simulink model "test_kalman_scaling"  (R2024a)
settings: Solver=FixedStepAuto  StartTime=0.0  StopTime=4e-4  FixedStep=8e-9  RelTol=1e-3
values from neighbouring files (symbols this model uses):
  A1 = [0,                  1,  0, 0,   0, 0 ... (first row only)    [three_axis_plant_ver_0_init.m]
  A2 = [0,                  1,  0, 0,   0, 0 ... (first row only)    [three_axis_plant_ver_0_init.m]
  B1 = [0; p.C_f/p.m; 0; p.C_f_xz/p.m; 0; p.C_f_xy/p.m;]    [three_axis_plant_ver_0_init.m]
  C1 = [p.C_el_x,  0,         p.C_el_xz,    0, p.C_el_xy, 0;       0,         p.C_el_x,          0,    0,         0, 0;       p.C_el_zx,        0,   p.C_el_z,    0,    p.C_el_zy, 0]    [three_axis_plant_ver_0_init.m]
  eff_fun = @(V) cos(eff_w.*V.^2)./(eff_m*V.^4 + eff_n) + eff_p    [three_axis_plant_ver_0_init.m]
  G1 = [0 0 0; 1/p.m 0 0; 0 0 0; 0 1/p.m 0; 0 0 0; 0 0 1/p.m]    [three_axis_plant_ver_0_init.m]
  t_off = 2*T_max +(t_on + 100*(2*pi/abs(p.Omega_ip)))    [three_axis_plant_ver_0_init.m]
  t_on = 0*2*T_max*0.01    [three_axis_plant_ver_0_init.m]
undefined symbols (not defined in the file or in its folder): clqr, k, lqg, p, xc7z020clg400
libraries: hdlSSR x61, hdlBasic x40, simulink x10, vmcUtilities x1
(part 1 of 2)
settings Model: Creator=berndorfer
settings DebuggingCC: UnconnectedInputMsg=warning  UnconnectedOutputMsg=warning  UnconnectedLineMsg=warning
settings ModelReferenceCC: EnableRefExpFcnMdlSchedulingChecks=on
settings RTWCC: GPUComputeCapability=3.5  DLArmComputeVersion=19.05

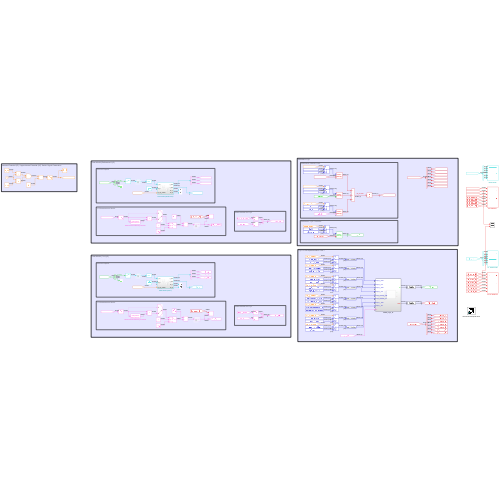
[thumbnail: Simulink's stored preview of the top-level diagram]
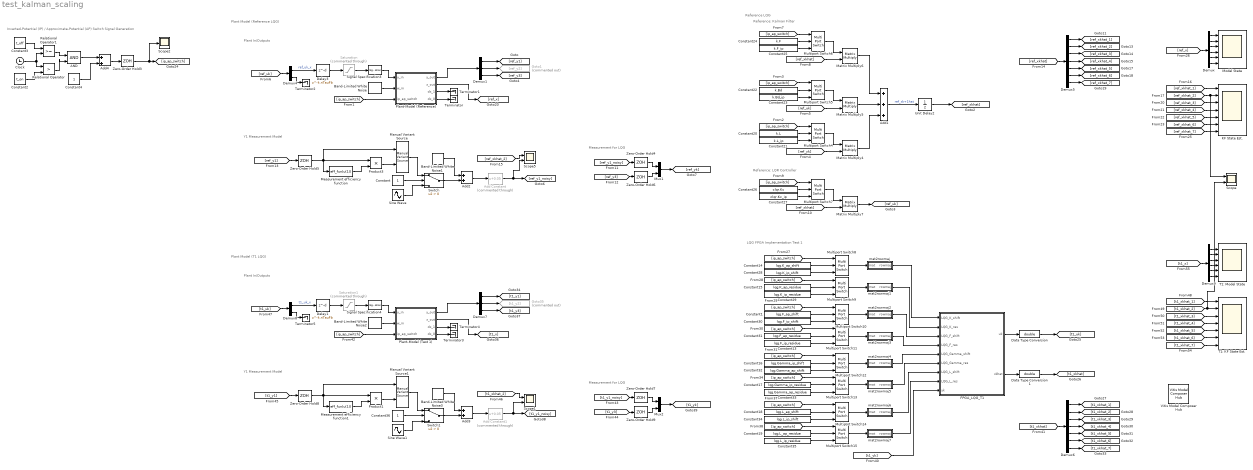
== system test_kalman_scaling ==
  note: LQG FPGA Implementation Test 1
  note: Plant In/Outputs
  note: Y1 Measurement Model
  note: Measurement for LQG
  note: Reference: LQR Controller
  note: Reference: Kalman Filter
  note: Reference LQG
  note: Plant Model (Reference LQG)
  note: Inverted-Potential (IP) / Approximate-Potential (AP) Switch Signal Generation
  note: Y1 Measurement Model
  note: Plant Model (T1 LQG)
  note: Plant In/Outputs
  note: Measurement for LQG
  AND : Logic  IconShape=distinctive  AllPortsSameDT=off  OutDataTypeStr=boolean
  Add Constant : Bias  Commented=through  Bias=0.05  SaturateOnIntegerOverflow=off
  Add Constant1 : Bias  Commented=through  Bias=0.05  SaturateOnIntegerOverflow=off
  Add1 : Sum  Inputs=+++
  Add2 : Sum
  Add3 : Sum
  Add4 : Sum
  Band-Limited White Noise : simulink/Sources/Band-Limited White Noise  Cov=P_W  Ts=p.Ts  seed=[23341; 896784; 46532]
  Band-Limited White Noise1 : simulink/Sources/Band-Limited White Noise  Cov=P_V  Ts=1/k.f_samp  seed=[73341]
  Band-Limited White Noise2 : simulink/Sources/Band-Limited White Noise  Cov=P_W  Ts=p.Ts  seed=[23341; 896784; 46532]
  Band-Limited White Noise3 : simulink/Sources/Band-Limited White Noise  Cov=P_V  Ts=1/k.f_samp  seed=[73341]
  Clock : Clock
  Constant : Constant
  Constant1 : Constant  Value=lqg.F_ap_shift  SampleTime=p.Ts
  Constant13 : Constant  Value=lqg.F_ip_residue  SampleTime=p.Ts
  Constant14 : Constant  Value=lqg.K_ap_shift  SampleTime=p.Ts
  Constant15 : Constant  Value=lqg.K_ap_residue  VectorParams1D=off  SampleTime=p.Ts
  Constant16 : Constant  Value=lqg.Gamma_ip_shift  SampleTime=p.Ts
  Constant17 : Constant  Value=lqg.Gamma_ip_residue  SampleTime=p.Ts
  Constant18 : Constant  Value=lqg.L_ap_shift  SampleTime=p.Ts
  Constant19 : Constant  Value=lqg.L_ap_residue  SampleTime=p.Ts
  Constant2 : Constant  Value=t_on
  Constant20 : Constant  Value=k.L  SampleTime=k.Ts
  Constant21 : Constant  Value=k.L_ip  SampleTime=k.Ts
  Constant22 : Constant  Value=k.Bd  SampleTime=k.Ts
  Constant23 : Constant  Value=k.Bd_ip  SampleTime=k.Ts
  Constant24 : Constant  Value=k.F  SampleTime=k.Ts
  Constant25 : Constant  Value=k.F_ip  SampleTime=k.Ts
  Constant26 : Constant  Value=clqr.Kc  SampleTime=k.Ts
  Constant27 : Constant  Value=clqr.Kc_ip  SampleTime=k.Ts
  Constant28 : Constant  Value=lqg.K_ip_shift  SampleTime=p.Ts
  Constant29 : Constant  Value=lqg.K_ip_residue  VectorParams1D=off  SampleTime=p.Ts
  Constant3 : Constant  Value=t_off
  Constant30 : Constant  Value=lqg.F_ip_shift  SampleTime=p.Ts
  Constant31 : Constant  Value=lqg.F_ap_residue  SampleTime=p.Ts
  Constant32 : Constant  Value=lqg.Gamma_ap_shift  SampleTime=p.Ts
  Constant33 : Constant  Value=lqg.Gamma_ap_residue  SampleTime=p.Ts
  Constant34 : Constant  Value=lqg.L_ip_shift  SampleTime=p.Ts
  Constant35 : Constant  Value=lqg.L_ip_residue  SampleTime=p.Ts
  Constant36 : Constant
  Constant4 : Constant
  Data Type Conversion : DataTypeConversion  OutDataTypeStr=double  SaturateOnIntegerOverflow=off  RndMeth=Floor
  Data Type Conversion1 : DataTypeConversion  OutDataTypeStr=double  SaturateOnIntegerOverflow=off  RndMeth=Floor
  Delay1 : Delay  DelayLength=k.nTauFb  SampleTime=k.Ts
  Delay3 : Delay  DelayLength=k.nTauFb  SampleTime=k.Ts
  Demux : Demux  Outputs=6
  Demux1 : Demux  Outputs=3
  Demux4 : Demux  Outputs=2
  Demux5 : Demux  Outputs=7
  Demux6 : Demux  Outputs=7
  Demux7 : Demux  Outputs=3
  Demux8 : Demux  Outputs=2
  Demux9 : Demux  Outputs=6
  FPGA_LQG_T1 : Subsystem
  Goto1 : Goto  Commented=on  GotoTag=ref_y2
  Goto35 : Goto  Commented=on  GotoTag=t1_y2
  KF State Est. : Scope  NumInputPorts=7
  Manual Variant Source : simulink/Signal Routing/Manual Variant Source  NumChoices=2  LabelModeActiveChoice=V_2
  Manual Variant Source1 : simulink/Signal Routing/Manual Variant Source  NumChoices=2  LabelModeActiveChoice=V_2
  Matrix Multiply{4..7} (4 alike) : Product  Multiplication=Matrix(*)
  Measurement efficiency function : MATLABFcn  MATLABFcn=eff_fun(u(1))
  Measurement efficiency function1 : MATLABFcn  MATLABFcn=eff_fun(u(1))
  Model State : Scope  NumInputPorts=6
  Multiport Switch{4..15} (12 alike) : MultiPortSwitch  Inputs=2  DiagnosticForDefault=Warning  SaturateOnIntegerOverflow=off  InputSameDT=off
  Mux1 : Mux  Inputs=2
  Mux2 : Mux  Inputs=2
  Plant-Model (Reference) : Subsystem
  Plant-Model (Test 1) : Subsystem
  Product1 : Product
  Product3 : Product
  Relational Operator : RelationalOperator  Operator=>  OutDataTypeStr=boolean  RndMeth=Simplest  InputSameDT=off
  Relational Operator1 : RelationalOperator  OutDataTypeStr=boolean  RndMeth=Simplest  InputSameDT=off
  Saturation : Saturate  Commented=through  UpperLimit=5  LowerLimit=-5
  Saturation1 : Saturate  Commented=through  UpperLimit=5  LowerLimit=-5
  Scope : Scope  NumInputPorts=2
  Scope1 : Scope  NumInputPorts=2
  Scope2 : Scope
  Scope5 : Scope  NumInputPorts=2
  Signal Specification3 : SignalSpecification  Dimensions=1
  Signal Specification4 : SignalSpecification  Dimensions=1
  Sine Wave : Sin  Amplitude=0.2  Frequency=2*pi*160e3  SampleTime=0
  Sine Wave1 : Sin  Amplitude=0.2  Frequency=2*pi*160e3  SampleTime=0
  Switch : Switch  Criteria=u2 > Threshold  SaturateOnIntegerOverflow=off  InputSameDT=off
  Switch1 : Switch  Criteria=u2 > Threshold  SaturateOnIntegerOverflow=off  InputSameDT=off
  T1: KF State Est. : Scope  NumInputPorts=7
  T1: Model State : Scope  NumInputPorts=6
  Terminator{,1..5} (6 alike) : Terminator
  Unit Delay2 : UnitDelay  InitialCondition=zeros(k.n_x,1)  SampleTime=k.Ts  HasFrameUpgradeWarning=on
  Vitis Model Composer Hub : vmcUtilities/Vitis Model Composer Hub  Tag=genX  CodeGeneration=off  SubsystemName=FPGA_LQG_T1  CompilationType=HDLCompilation  SubsystemType=HDLNode  ExportTypeV2=IP Catalog  StartColumn=1  NumberOfColumns=1  TargetDirectory=./netlist_lqg_t1  exportDesign=on  analyzeDesign=off  validateDesignOnHw=off  ExportType=AI Engines  IpVendor=xilinx.com  IpLibrary=hls  IpVersion=1.0  IpHWLanguage=Verilog  AieCompilerOptions={}  AieSimulatorOptions={}  CreateTestbench=off  TestbenchStackSize=10  RunRtlSim=off  RunCSim=off  RunAieSim=off  AieSimTimeout=50000  RunAieSimProfiling=off  LaunchVitisAnalyzer=off  PlotOutput=off  RunX86Sim=off  X86SimTimeout=10  GenHwImage=off  GenLibadfXo=on  GenHwValidationCode=off  PlatformType=Not Specified  HwSystemType=Baremetal  HwValidationTarget=hw  ProjDevice=xc7z020clg400-2  ProjDevicePart=xc7z020clg400-2  AIEType=None  SamplePeriod=-1  ClockFrequency=200  DataPathParallelism=1  xilinxfamily=zynq  part=xc7z020  speed=-2  package=clg400  directory=./code/ip/FPGA_LQG_T1/src  testbench=off  incr_netlist=off  synthesis_tool=Vivado  clock_wrapper=Clock Enables  dbl_ovrd=According to Block Masks  dcm_input_clock_period=10  sysclk_period=64  simulink_period=64e-9  eval_field=0  IPInfoJsonString="{\"DUTSubsystemName\":\"FPGA_LQG_T1\",\"HDLSubsystem\":{\"SubsystemName\":\"FPGA_LQG_T1\",\"IPName\":\"FPGA_LQG_Scaling_Test\",\"IPLibrary\":\"VMC\",\"IPVendor\":\"ACIN\",\"IPVersion\":\"1.0\",\"TargetDirectory\":\"./netlist_lqg_t1\",\"SubsystemDir\":\"./netlist_lqg_t1/ip/FPGA_LQG_T1\",\"FreqHz\":\"15625000\"},\"SubsystemTag\":\"HDLNode\"}"  LogFileName=/home/user/host_home/work/acin/projects/universal_lqg/lqg-fp7-firmware/matlab/netlist_lqg_t1/model_composer.log  NThreads=4  IPConfigFile=/tmp/vmctmp-user/13/ipconfig.json
  Zero-Order Hold3 : ZeroOrderHold  SampleTime=p.Ts
  Zero-Order Hold{4,6..7,9} (4 alike) : ZeroOrderHold  SampleTime=1/k.f_samp
  Zero-Order Hold5 : ZeroOrderHold  SampleTime=p.Ts
  Zero-Order Hold8 : ZeroOrderHold  SampleTime=p.Ts
  mat2rowmaj : Subsystem
  mat2rowmaj1 : Subsystem
  mat2rowmaj2 : Subsystem
  mat2rowmaj3 : Subsystem
  mat2rowmaj4 : Subsystem
  mat2rowmaj5 : Subsystem
  mat2rowmaj6 : Subsystem
  mat2rowmaj7 : Subsystem
  wires:
  Band-Limited White Noise/1 -> Plant-Model (Reference)/2(w_in)
  [ip_ap_switch] -> Plant-Model (Reference)/3(ip_ap_switch)
  AND/1 -> Add4/1
  Constant2/1 -> Relational Operator/2
  Clock/1 -> Relational Operator/1, Relational Operator1/2
  Relational Operator1/1 -> AND/1
  Add4/1 -> Zero-Order Hold3/1
  Relational Operator/1 -> AND/2
  Constant3/1 -> Relational Operator1/1
  Constant4/1 -> Add4/2
  Plant-Model (Reference)/1(y_out) -> Demux1/1
  Demux1/3 -> [ref_y3]
  Demux1/1 -> [ref_y1]
  Plant-Model (Reference)/2(x_out) -> [ref_x]
  Measurement efficiency function/1 -> Product3/2
  Sine Wave/1 -> Switch/3
  Switch/1 -> Add2/2
  Product3/1 -> Manual Variant Source/2
  Add2/1 -> Add Constant/1
  Constant/1 -> Switch/2
  Band-Limited White Noise1/1 -> Add2/1
  Add Constant/1 -> Scope5/2, [ref_y1_noisy]
  Zero-Order Hold5/1 -> Measurement efficiency function/1, Manual Variant Source/1, Product3/1
  [ref_y1] -> Zero-Order Hold5/1
  Signal Specification3/1 -> Plant-Model (Reference)/1(u_in)
  Saturation/1 -> Signal Specification3/1
  Delay3/1 -> Saturation/1
  Demux4/1 -> Delay3/1  "ref_uk_x"
  Demux1/2 -> Goto1/1
  Zero-Order Hold3/1 -> Scope2/1, [ip_ap_switch]
  Plant-Model (Reference)/4(dx_0) -> Terminator/1
  Plant-Model (Reference)/3(dx_1) -> Terminator1/1
  Constant20/1 -> Multiport Switch4/2
  [ip_ap_switch] -> Multiport Switch4/1
  Constant21/1 -> Multiport Switch4/3
  [ip_ap_switch] -> Multiport Switch5/1
  Constant22/1 -> Multiport Switch5/2
  Constant23/1 -> Multiport Switch5/3
  Multiport Switch4/1 -> Matrix Multiply4/1
  [ref_yk] -> Matrix Multiply4/2
  Multiport Switch5/1 -> Matrix Multiply5/1
  [ref_uk] -> Matrix Multiply5/2
  Constant24/1 -> Multiport Switch6/2
  Constant25/1 -> Multiport Switch6/3
  Multiport Switch6/1 -> Matrix Multiply6/1
  [ip_ap_switch] -> Multiport Switch6/1
  [ref_xkhat] -> Matrix Multiply6/2
  Matrix Multiply5/1 -> Add1/2
  Matrix Multiply6/1 -> Add1/1
  Matrix Multiply4/1 -> Add1/3
  Add1/1 -> Unit Delay2/1  "ref_xk+1hat"
  Unit Delay2/1 -> [ref_xkhat]
  Demux4/2 -> Terminator2/1
  [ref_uk] -> Demux4/1
  Constant26/1 -> Multiport Switch7/2
  Constant27/1 -> Multiport Switch7/3
  [ip_ap_switch] -> Multiport Switch7/1
  Multiport Switch7/1 -> Matrix Multiply7/1
  [ref_xkhat] -> Matrix Multiply7/2
  Matrix Multiply7/1 -> [ref_uk]
  [ref_y1_noisy] -> Zero-Order Hold4/1
  [ref_y3] -> Zero-Order Hold6/1
  Zero-Order Hold4/1 -> Mux1/1
  Zero-Order Hold6/1 -> Mux1/2
  Mux1/1 -> [ref_yk]
  Manual Variant Source/1 -> Switch/1
  [ref_xkhat] -> Demux5/1
  Demux5/1 -> [ref_xkhat_1]
  Demux5/2 -> [ref_xkhat_2]
  Demux5/3 -> [ref_xkhat_3]
  Demux5/4 -> [ref_xkhat_4]
  Demux5/5 -> [ref_xkhat_5]
  Demux5/6 -> [ref_xkhat_6]
  Demux5/7 -> [ref_xkhat_7]
  [ref_xkhat_2] -> Scope5/1
  [ref_xkhat_1] -> KF State Est./1
  [ref_xkhat_2] -> Scope/1, KF State Est./2
  [ref_xkhat_3] -> KF State Est./3
  [ref_xkhat_4] -> KF State Est./4
  [ref_xkhat_5] -> KF State Est./5
  [ref_xkhat_6] -> KF State Est./6
  [ref_xkhat_7] -> KF State Est./7
  Demux/5 -> Model State/5
  Demux/4 -> Model State/4
  Demux/1 -> Model State/1
  Demux/3 -> Model State/3
  Demux/2 -> Model State/2
  Demux/6 -> Model State/6
  [ref_x] -> Demux/1
  Constant14/1 -> Multiport Switch8/2
  Constant28/1 -> Multiport Switch8/3
  Multiport Switch8/1 -> mat2rowmaj/1(mat)
  [ip_ap_switch] -> Multiport Switch8/1
  [ip_ap_switch] -> Multiport Switch9/1
  Constant15/1 -> Multiport Switch9/2
  Constant29/1 -> Multiport Switch9/3
  Multiport Switch9/1 -> mat2rowmaj1/1(mat)
  [ip_ap_switch] -> Multiport Switch10/1
  Constant1/1 -> Multiport Switch10/2
  [ip_ap_switch] -> Multiport Switch11/1
  Constant31/1 -> Multiport Switch11/2
  Constant30/1 -> Multiport Switch10/3
  Constant13/1 -> Multiport Switch11/3
  Multiport Switch11/1 -> mat2rowmaj3/1(mat)
  Multiport Switch10/1 -> mat2rowmaj2/1(mat)
  [ip_ap_switch] -> Multiport Switch13/1
  Constant16/1 -> Multiport Switch12/2
  Constant32/1 -> Multiport Switch12/3
  Constant33/1 -> Multiport Switch13/3
  [ip_ap_switch] -> Multiport Switch12/1
  Constant17/1 -> Multiport Switch13/2
  Multiport Switch12/1 -> mat2rowmaj4/1(mat)
  Multiport Switch13/1 -> mat2rowmaj5/1(mat)
  Constant34/1 -> Multiport Switch14/3
  Constant35/1 -> Multiport Switch15/3
  Constant19/1 -> Multiport Switch15/2
  Constant18/1 -> Multiport Switch14/2
  [ip_ap_switch] -> Multiport Switch15/1
  [ip_ap_switch] -> Multiport Switch14/1
  Multiport Switch14/1 -> mat2rowmaj6/1(mat)
  Multiport Switch15/1 -> mat2rowmaj7/1(mat)
  [t1_yk] -> FPGA_LQG_T1/9(yk)
  mat2rowmaj7/1(rowmaj) -> FPGA_LQG_T1/8(LQG_L_res)
  mat2rowmaj6/1(rowmaj) -> FPGA_LQG_T1/7(LQG_L_shift)
  mat2rowmaj/1(rowmaj) -> FPGA_LQG_T1/1(LQG_K_shift)
  mat2rowmaj1/1(rowmaj) -> FPGA_LQG_T1/2(LQG_K_res)
  mat2rowmaj2/1(rowmaj) -> FPGA_LQG_T1/3(LQG_F_shift)
  mat2rowmaj4/1(rowmaj) -> FPGA_LQG_T1/5(LQG_Gamma_shift)
  mat2rowmaj5/1(rowmaj) -> FPGA_LQG_T1/6(LQG_Gamma_res)
  mat2rowmaj3/1(rowmaj) -> FPGA_LQG_T1/4(LQG_F_res)
  FPGA_LQG_T1/1(uk) -> Data Type Conversion/1
  FPGA_LQG_T1/2(xkhat) -> Data Type Conversion1/1
  Demux6/7 -> [t1_xkhat_7]
  Demux6/6 -> [t1_xkhat_6]
  Demux6/3 -> [t1_xkhat_3]
  Demux6/5 -> [t1_xkhat_5]
  [t1_xkhat] -> Demux6/1
  Demux6/2 -> [t1_xkhat_2]
  Demux6/1 -> [t1_xkhat_1]
  Demux6/4 -> [t1_xkhat_4]
  Signal Specification4/1 -> Plant-Model (Test 1)/1(u_in)
  [t1_y1] -> Zero-Order Hold8/1
  [t1_uk] -> Demux8/1
  Mux2/1 -> [t1_yk]
  Add Constant1/1 -> Scope1/2, [t1_y1_noisy]
  Plant-Model (Test 1)/3(dx_1) -> Terminator4/1
  Switch1/1 -> Add3/2
  Sine Wave1/1 -> Switch1/3
  Plant-Model (Test 1)/1(y_out) -> Demux7/1
  Demux7/3 -> [t1_y3]
  Saturation1/1 -> Signal Specification4/1
  Demux7/1 -> [t1_y1]
  Demux7/2 -> Goto35/1
  [t1_y1_noisy] -> Zero-Order Hold7/1
  [t1_y3] -> Zero-Order Hold9/1
  Plant-Model (Test 1)/2(x_out) -> [t1_x]
  Constant36/1 -> Switch1/2
  Zero-Order Hold7/1 -> Mux2/1
  Zero-Order Hold9/1 -> Mux2/2
  Measurement efficiency function1/1 -> Product1/2
  [t1_xkhat_2] -> Scope1/1
  Band-Limited White Noise2/1 -> Plant-Model (Test 1)/2(w_in)
  Zero-Order Hold8/1 -> Measurement efficiency function1/1, Manual Variant Source1/1, Product1/1
  [ip_ap_switch] -> Plant-Model (Test 1)/3(ip_ap_switch)
  Demux8/2 -> Terminator5/1
  Plant-Model (Test 1)/4(dx_0) -> Terminator3/1
  Demux8/1 -> Delay1/1  "t1_uk_x"
  Product1/1 -> Manual Variant Source1/2
  Add3/1 -> Add Constant1/1
  Band-Limited White Noise3/1 -> Add3/1
  Delay1/1 -> Saturation1/1
  Manual Variant Source1/1 -> Switch1/1
  Demux9/3 -> T1: Model State/3
  [t1_xkhat_4] -> T1: KF State Est./4
  Demux9/2 -> T1: Model State/2
  [t1_xkhat_5] -> T1: KF State Est./5
  [t1_xkhat_7] -> T1: KF State Est./7
  [t1_x] -> Demux9/1
  [t1_xkhat_3] -> T1: KF State Est./3
  Demux9/6 -> T1: Model State/6
  [t1_xkhat_6] -> T1: KF State Est./6
  [t1_xkhat_1] -> T1: KF State Est./1
  [t1_xkhat_2] -> Scope/2, T1: KF State Est./2
  Demux9/1 -> T1: Model State/1
  Demux9/4 -> T1: Model State/4
  Demux9/5 -> T1: Model State/5
  Data Type Conversion/1 -> [t1_uk]
  Data Type Conversion1/1 -> [t1_xkhat]

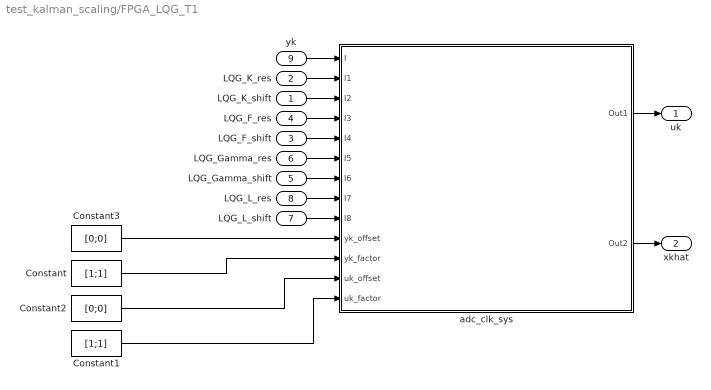
== system test_kalman_scaling/FPGA_LQG_T1 ==
  LQG_K_shift : Inport
  LQG_K_res : Inport  Port=2
  LQG_F_shift : Inport  Port=3
  LQG_F_res : Inport  Port=4
  LQG_Gamma_shift : Inport  Port=5
  LQG_Gamma_res : Inport  Port=6
  LQG_L_shift : Inport  Port=7
  LQG_L_res : Inport  Port=8
  yk : Inport  Port=9
  Constant : Constant  Value=[1;1]  SampleTime=8e-9
  Constant1 : Constant  Value=[1;1]  SampleTime=8e-9
  Constant2 : Constant  Value=[0;0]  SampleTime=8e-9
  Constant3 : Constant  Value=[0;0]  SampleTime=8e-9
  adc_clk_sys : Subsystem
  uk : Outport
  xkhat : Outport  Port=2
  wires:
  yk/1 -> adc_clk_sys/1(I)
  LQG_K_res/1 -> adc_clk_sys/2(I1)
  LQG_K_shift/1 -> adc_clk_sys/3(I2)
  LQG_F_res/1 -> adc_clk_sys/4(I3)
  LQG_F_shift/1 -> adc_clk_sys/5(I4)
  LQG_Gamma_res/1 -> adc_clk_sys/6(I5)
  LQG_Gamma_shift/1 -> adc_clk_sys/7(I6)
  LQG_L_res/1 -> adc_clk_sys/8(I7)
  LQG_L_shift/1 -> adc_clk_sys/9(I8)
  adc_clk_sys/1(Out1) -> uk/1
  adc_clk_sys/2(Out2) -> xkhat/1
  Constant3/1 -> adc_clk_sys/10(yk_offset)
  Constant/1 -> adc_clk_sys/11(yk_factor)
  Constant2/1 -> adc_clk_sys/12(uk_offset)
  Constant1/1 -> adc_clk_sys/13(uk_factor)

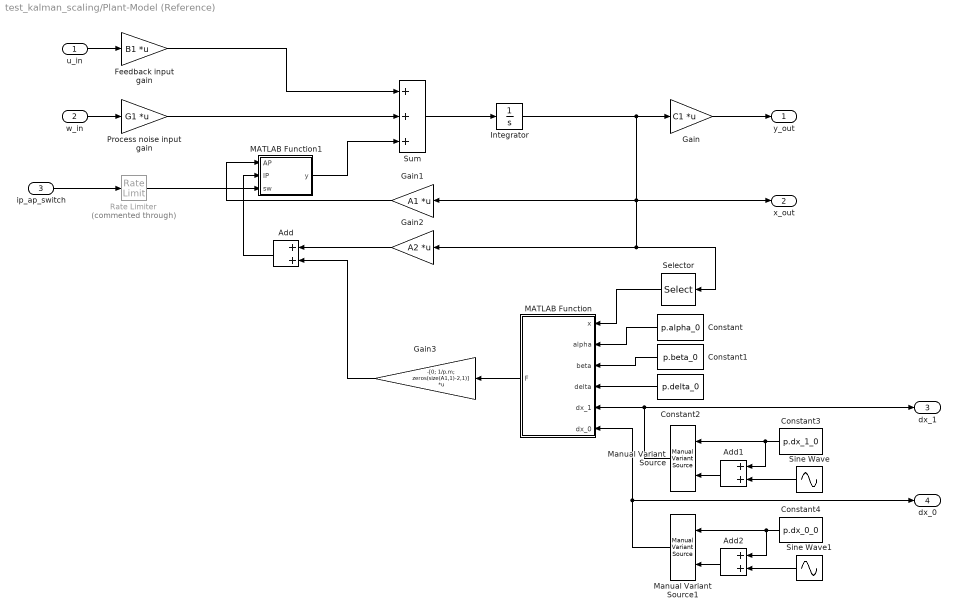
== system test_kalman_scaling/Plant-Model (Reference) ==
  u_in : Inport
  w_in : Inport  Port=2
  ip_ap_switch : Inport  Port=3
  Add : Sum
  Add1 : Sum
  Add2 : Sum
  Constant : Constant  Value=p.alpha_0
  Constant1 : Constant  Value=p.beta_0
  Constant2 : Constant  Value=p.delta_0
  Constant3 : Constant  Value=p.dx_1_0
  Constant4 : Constant  Value=p.dx_0_0
  Feedback input gain : Gain  Gain=B1  Multiplication=Matrix(K*u)
  Gain : Gain  Gain=C1  Multiplication=Matrix(K*u)
  Gain1 : Gain  Gain=A1  Multiplication=Matrix(K*u)
  Gain2 : Gain  Gain=A2  Multiplication=Matrix(K*u)
  Gain3 : Gain  Gain=-[0; 1/p.m; zeros(size(A1,1)-2,1)]  Multiplication=Matrix(K*u)
  Integrator : Integrator  InitialCondition=zeros(size(A1,1),1)
  MATLAB Function : MATLAB Function  TreatAsAtomicUnit=on
  MATLAB Function1 : MATLAB Function  TreatAsAtomicUnit=on
  Manual Variant Source : simulink/Signal Routing/Manual Variant Source  NumChoices=2  LabelModeActiveChoice=V_2
  Manual Variant Source1 : simulink/Signal Routing/Manual Variant Source  NumChoices=2  LabelModeActiveChoice=V_1
  Process noise input gain : Gain  Gain=G1  Multiplication=Matrix(K*u)
  Rate Limiter : RateLimiter  Commented=through  RisingSlewLimit=1/(100*k.Ts)  FallingSlewLimit=-1/(100*k.Ts)  SampleTimeMode=inherited  InitialCondition=2
  Selector : Selector  InputPortWidth=size(A1,1)  IndexOptions=Index vector (dialog)  Indices=[1]  OutputSizes=1
  Sine Wave : Sin  Amplitude=6e-9  Bias=0e-9  Frequency=100*2*pi  SampleTime=0
  Sine Wave1 : Sin  Amplitude=2e-9  Bias=0e-9  Frequency=100*2*pi  SampleTime=0
  Sum : Sum  Inputs=+++
  y_out : Outport
  x_out : Outport  Port=2
  dx_1 : Outport  Port=3
  dx_0 : Outport  Port=4
  wires:
  w_in/1 -> Process noise input gain/1
  u_in/1 -> Feedback input gain/1
  Sum/1 -> Integrator/1
  Feedback input gain/1 -> Sum/1
  Process noise input gain/1 -> Sum/2
  Integrator/1 -> Gain/1, x_out/1, Gain2/1, Selector/1, Gain1/1
  Selector/1 -> MATLAB Function/1(x)
  Gain/1 -> y_out/1
  MATLAB Function1/1(y) -> Sum/3
  Gain1/1 -> MATLAB Function1/1(AP)
  ip_ap_switch/1 -> Rate Limiter/1
  Rate Limiter/1 -> MATLAB Function1/3(sw)
  MATLAB Function/1(F) -> Gain3/1
  Add/1 -> MATLAB Function1/2(IP)
  Gain2/1 -> Add/1
  Constant/1 -> MATLAB Function/2(alpha)
  Constant1/1 -> MATLAB Function/3(beta)
  Constant2/1 -> MATLAB Function/4(delta)
  Manual Variant Source/1 -> MATLAB Function/5(dx_1), dx_1/1
  Manual Variant Source1/1 -> dx_0/1, MATLAB Function/6(dx_0)
  Constant3/1 -> Add1/1, Manual Variant Source/1
  Constant4/1 -> Add2/1, Manual Variant Source1/1
  Add1/1 -> Manual Variant Source/2
  Add2/1 -> Manual Variant Source1/2
  Sine Wave/1 -> Add1/2
  Sine Wave1/1 -> Add2/2
  Gain3/1 -> Add/2

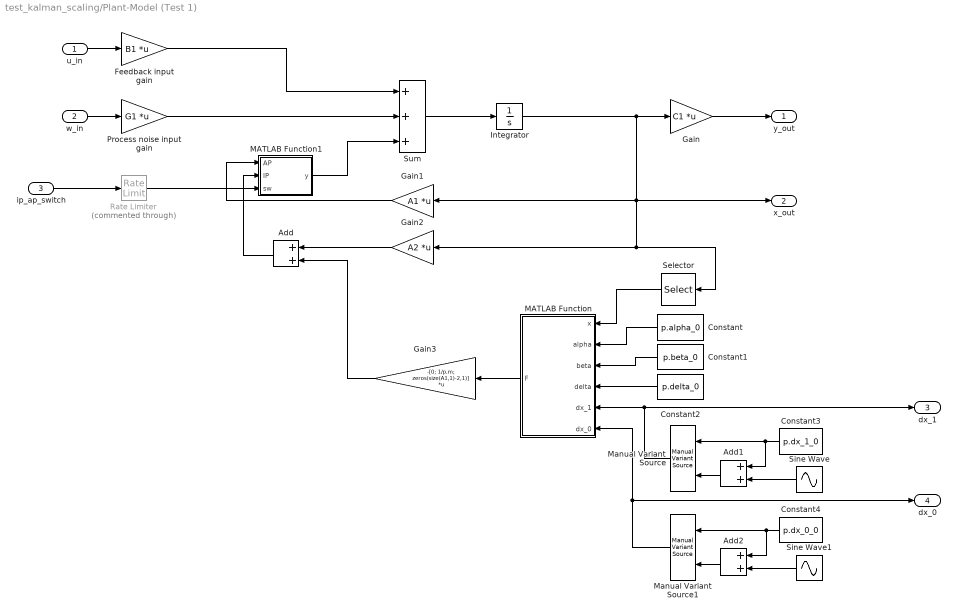
== system test_kalman_scaling/Plant-Model (Test 1) ==
  u_in : Inport
  w_in : Inport  Port=2
  ip_ap_switch : Inport  Port=3
  Add : Sum
  Add1 : Sum
  Add2 : Sum
  Constant : Constant  Value=p.alpha_0
  Constant1 : Constant  Value=p.beta_0
  Constant2 : Constant  Value=p.delta_0
  Constant3 : Constant  Value=p.dx_1_0
  Constant4 : Constant  Value=p.dx_0_0
  Feedback input gain : Gain  Gain=B1  Multiplication=Matrix(K*u)
  Gain : Gain  Gain=C1  Multiplication=Matrix(K*u)
  Gain1 : Gain  Gain=A1  Multiplication=Matrix(K*u)
  Gain2 : Gain  Gain=A2  Multiplication=Matrix(K*u)
  Gain3 : Gain  Gain=-[0; 1/p.m; zeros(size(A1,1)-2,1)]  Multiplication=Matrix(K*u)
  Integrator : Integrator  InitialCondition=zeros(size(A1,1),1)
  MATLAB Function : MATLAB Function  TreatAsAtomicUnit=on
  MATLAB Function1 : MATLAB Function  TreatAsAtomicUnit=on
  Manual Variant Source : simulink/Signal Routing/Manual Variant Source  NumChoices=2  LabelModeActiveChoice=V_2
  Manual Variant Source1 : simulink/Signal Routing/Manual Variant Source  NumChoices=2  LabelModeActiveChoice=V_1
  Process noise input gain : Gain  Gain=G1  Multiplication=Matrix(K*u)
  Rate Limiter : RateLimiter  Commented=through  RisingSlewLimit=1/(100*k.Ts)  FallingSlewLimit=-1/(100*k.Ts)  SampleTimeMode=inherited  InitialCondition=2
  Selector : Selector  InputPortWidth=size(A1,1)  IndexOptions=Index vector (dialog)  Indices=[1]  OutputSizes=1
  Sine Wave : Sin  Amplitude=6e-9  Bias=0e-9  Frequency=100*2*pi  SampleTime=0
  Sine Wave1 : Sin  Amplitude=2e-9  Bias=0e-9  Frequency=100*2*pi  SampleTime=0
  Sum : Sum  Inputs=+++
  y_out : Outport
  x_out : Outport  Port=2
  dx_1 : Outport  Port=3
  dx_0 : Outport  Port=4
  wires:
  w_in/1 -> Process noise input gain/1
  u_in/1 -> Feedback input gain/1
  Sum/1 -> Integrator/1
  Feedback input gain/1 -> Sum/1
  Process noise input gain/1 -> Sum/2
  Integrator/1 -> Gain/1, x_out/1, Gain2/1, Selector/1, Gain1/1
  Selector/1 -> MATLAB Function/1(x)
  Gain/1 -> y_out/1
  MATLAB Function1/1(y) -> Sum/3
  Gain1/1 -> MATLAB Function1/1(AP)
  ip_ap_switch/1 -> Rate Limiter/1
  Rate Limiter/1 -> MATLAB Function1/3(sw)
  MATLAB Function/1(F) -> Gain3/1
  Add/1 -> MATLAB Function1/2(IP)
  Gain2/1 -> Add/1
  Constant/1 -> MATLAB Function/2(alpha)
  Constant1/1 -> MATLAB Function/3(beta)
  Constant2/1 -> MATLAB Function/4(delta)
  Manual Variant Source/1 -> MATLAB Function/5(dx_1), dx_1/1
  Manual Variant Source1/1 -> dx_0/1, MATLAB Function/6(dx_0)
  Constant3/1 -> Add1/1, Manual Variant Source/1
  Constant4/1 -> Add2/1, Manual Variant Source1/1
  Add1/1 -> Manual Variant Source/2
  Add2/1 -> Manual Variant Source1/2
  Sine Wave/1 -> Add1/2
  Sine Wave1/1 -> Add2/2
  Gain3/1 -> Add/2

== system test_kalman_scaling/mat2rowmaj ==
  mat : Inport
  Reshape1 : Reshape
  Transpose1 : Math  Operator=transpose
  rowmaj : Outport
  wires:
  Reshape1/1 -> rowmaj/1
  Transpose1/1 -> Reshape1/1
  mat/1 -> Transpose1/1

== system test_kalman_scaling/mat2rowmaj1 ==
  mat : Inport
  Reshape1 : Reshape
  Transpose1 : Math  Operator=transpose
  rowmaj : Outport
  wires:
  Reshape1/1 -> rowmaj/1
  Transpose1/1 -> Reshape1/1
  mat/1 -> Transpose1/1

== system test_kalman_scaling/mat2rowmaj2 ==
  mat : Inport
  Reshape1 : Reshape
  Transpose1 : Math  Operator=transpose
  rowmaj : Outport
  wires:
  Reshape1/1 -> rowmaj/1
  Transpose1/1 -> Reshape1/1
  mat/1 -> Transpose1/1

== system test_kalman_scaling/mat2rowmaj3 ==
  mat : Inport
  Reshape1 : Reshape
  Transpose1 : Math  Operator=transpose
  rowmaj : Outport
  wires:
  Reshape1/1 -> rowmaj/1
  Transpose1/1 -> Reshape1/1
  mat/1 -> Transpose1/1

== system test_kalman_scaling/mat2rowmaj4 ==
  mat : Inport
  Reshape1 : Reshape
  Transpose1 : Math  Operator=transpose
  rowmaj : Outport
  wires:
  Reshape1/1 -> rowmaj/1
  Transpose1/1 -> Reshape1/1
  mat/1 -> Transpose1/1

== system test_kalman_scaling/mat2rowmaj5 ==
  mat : Inport
  Reshape1 : Reshape
  Transpose1 : Math  Operator=transpose
  rowmaj : Outport
  wires:
  Reshape1/1 -> rowmaj/1
  Transpose1/1 -> Reshape1/1
  mat/1 -> Transpose1/1

== system test_kalman_scaling/mat2rowmaj6 ==
  mat : Inport
  Reshape1 : Reshape
  Transpose1 : Math  Operator=transpose
  rowmaj : Outport
  wires:
  Reshape1/1 -> rowmaj/1
  Transpose1/1 -> Reshape1/1
  mat/1 -> Transpose1/1

== system test_kalman_scaling/mat2rowmaj7 ==
  mat : Inport
  Reshape1 : Reshape
  Transpose1 : Math  Operator=transpose
  rowmaj : Outport
  wires:
  Reshape1/1 -> rowmaj/1
  Transpose1/1 -> Reshape1/1
  mat/1 -> Transpose1/1

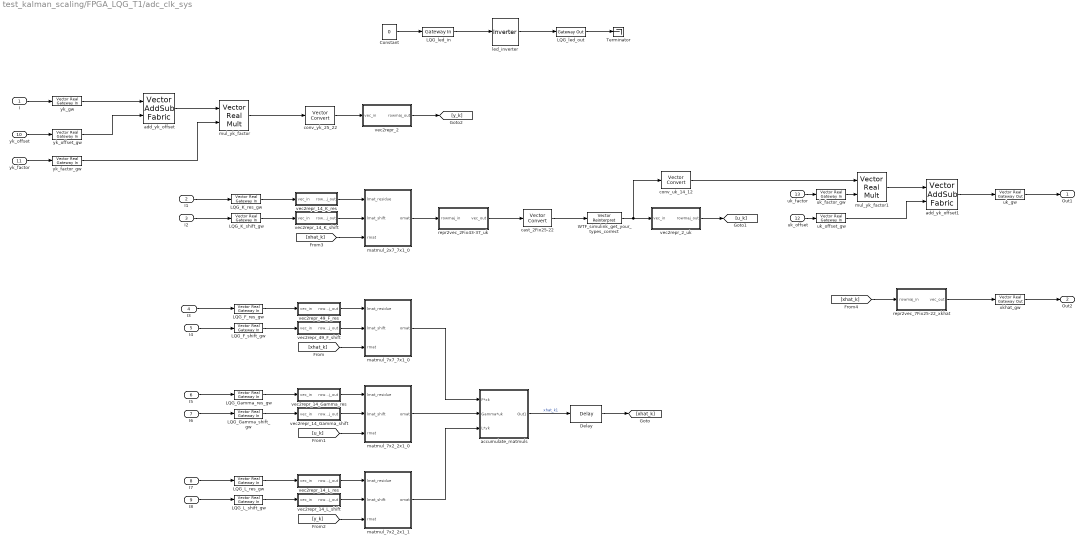
== system test_kalman_scaling/FPGA_LQG_T1/adc_clk_sys ==
  I : Inport
  I1 : Inport  Port=2
  I2 : Inport  Port=3
  I3 : Inport  Port=4
  I4 : Inport  Port=5
  I5 : Inport  Port=6
  I6 : Inport  Port=7
  I7 : Inport  Port=8
  I8 : Inport  Port=9
  yk_offset : Inport  Port=10
  yk_factor : Inport  Port=11
  uk_offset : Inport  Port=12
  uk_factor : Inport  Port=13
  Constant : Constant  Value=0
  Delay : hdlBasic/Delay  rst=off  en=off  latency=1  reg_retiming=off  XmcBlockStatus=1  maskContainerNames=group1  block_type=delay  block_config=sysgen:Delay_config
  LQG_F_res_gw : hdlSSR/Vector Real Gateway In  gui_display_data_type=Fixed-point  arith_type=Signed (2's comp)  n_bits=18  bin_pt=14  preci_type=Single  exp_width=8  frac_width=24  quantization="Round  (unbiased: +/- Inf)"  overflow=Saturate  period=k.Ts  sg_ssr=7*7  UseAsADC=off  ADCChannel='1'  interface=None  automatic_assignment=on  address_offset=hex2dec('00')  intf_name=''  intf_description=''  default_value=0  timing_constraint=None  locs_specified=off  LOCs={}  io_standard={}  inherit_from_input=off  hdl_port=on  interface_prev=1  block_type=realgatewayin_ssr  XmcBlockStatus=1  sg_ssr_prev=49  maskContainerNames=group4  block_width_w=590  block_height_w=670  block_width=640  block_height=850
  LQG_F_shift_gw : hdlSSR/Vector Real Gateway In  gui_display_data_type=Fixed-point  arith_type=Unsigned  n_bits=5  bin_pt=0  preci_type=Single  exp_width=8  frac_width=24  quantization="Round  (unbiased: +/- Inf)"  overflow=Saturate  period=k.Ts  sg_ssr=7*7  UseAsADC=off  ADCChannel='1'  interface=None  automatic_assignment=on  address_offset=hex2dec('00')  intf_name=''  intf_description=''  default_value=0  timing_constraint=None  locs_specified=off  LOCs={}  io_standard={}  inherit_from_input=off  hdl_port=on  interface_prev=1  block_type=realgatewayin_ssr  XmcBlockStatus=1  sg_ssr_prev=49  maskContainerNames=group4  block_width_w=590  block_height_w=670  block_width=640  block_height=850
  LQG_Gamma_res_gw : hdlSSR/Vector Real Gateway In  gui_display_data_type=Fixed-point  arith_type=Signed (2's comp)  n_bits=18  bin_pt=14  preci_type=Single  exp_width=8  frac_width=24  quantization="Round  (unbiased: +/- Inf)"  overflow=Saturate  period=k.Ts  sg_ssr=7*2  UseAsADC=off  ADCChannel='1'  interface=None  automatic_assignment=on  address_offset=hex2dec('00')  intf_name=''  intf_description=''  default_value=0  timing_constraint=None  locs_specified=off  LOCs={}  io_standard={}  inherit_from_input=off  hdl_port=on  interface_prev=1  block_type=realgatewayin_ssr  XmcBlockStatus=1  sg_ssr_prev=14  maskContainerNames=group4  block_width_w=590  block_height_w=670  block_width=640  block_height=850
  LQG_Gamma_shift_gw : hdlSSR/Vector Real Gateway In  gui_display_data_type=Fixed-point  arith_type=Unsigned  n_bits=5  bin_pt=0  preci_type=Single  exp_width=8  frac_width=24  quantization="Round  (unbiased: +/- Inf)"  overflow=Saturate  period=k.Ts  sg_ssr=7*2  UseAsADC=off  ADCChannel='1'  interface=None  automatic_assignment=on  address_offset=hex2dec('00')  intf_name=''  intf_description=''  default_value=0  timing_constraint=None  locs_specified=off  LOCs={}  io_standard={}  inherit_from_input=off  hdl_port=on  interface_prev=1  block_type=realgatewayin_ssr  XmcBlockStatus=1  sg_ssr_prev=14  maskContainerNames=group4  block_width_w=590  block_height_w=670  block_width=640  block_height=850
  LQG_K_res_gw : hdlSSR/Vector Real Gateway In  gui_display_data_type=Fixed-point  arith_type=Signed (2's comp)  n_bits=18  bin_pt=14  preci_type=Single  exp_width=8  frac_width=24  quantization="Round  (unbiased: +/- Inf)"  overflow=Saturate  period=k.Ts  sg_ssr=2*7  UseAsADC=off  ADCChannel='1'  interface=None  automatic_assignment=on  address_offset=hex2dec('00')  intf_name=''  intf_description=''  default_value=0  timing_constraint=None  locs_specified=off  LOCs={}  io_standard={}  inherit_from_input=off  hdl_port=on  interface_prev=1  block_type=realgatewayin_ssr  XmcBlockStatus=1  sg_ssr_prev=14  maskContainerNames=group4  block_width_w=590  block_height_w=670  block_width=640  block_height=850
  LQG_K_shift_gw : hdlSSR/Vector Real Gateway In  gui_display_data_type=Fixed-point  arith_type=Signed (2's comp)  n_bits=6  bin_pt=0  preci_type=Single  exp_width=8  frac_width=24  quantization="Round  (unbiased: +/- Inf)"  overflow=Saturate  period=k.Ts  sg_ssr=2*7  UseAsADC=off  ADCChannel='1'  interface=None  automatic_assignment=on  address_offset=hex2dec('00')  intf_name=''  intf_description=''  default_value=0  timing_constraint=None  locs_specified=off  LOCs={}  io_standard={}  inherit_from_input=off  hdl_port=on  interface_prev=1  block_type=realgatewayin_ssr  XmcBlockStatus=1  sg_ssr_prev=14  maskContainerNames=group4  block_width_w=590  block_height_w=670  block_width=640  block_height=850
  LQG_L_res_gw : hdlSSR/Vector Real Gateway In  gui_display_data_type=Fixed-point  arith_type=Signed (2's comp)  n_bits=18  bin_pt=14  preci_type=Single  exp_width=8  frac_width=24  quantization="Round  (unbiased: +/- Inf)"  overflow=Saturate  period=k.Ts  sg_ssr=7*2  UseAsADC=off  ADCChannel='1'  interface=None  automatic_assignment=on  address_offset=hex2dec('00')  intf_name=''  intf_description=''  default_value=0  timing_constraint=None  locs_specified=off  LOCs={}  io_standard={}  inherit_from_input=off  hdl_port=on  interface_prev=1  block_type=realgatewayin_ssr  XmcBlockStatus=1  sg_ssr_prev=14  maskContainerNames=group4  block_width_w=590  block_height_w=670  block_width=640  block_height=850
  LQG_L_shift_gw : hdlSSR/Vector Real Gateway In  gui_display_data_type=Fixed-point  arith_type=Unsigned  n_bits=5  bin_pt=0  preci_type=Single  exp_width=8  frac_width=24  quantization="Round  (unbiased: +/- Inf)"  overflow=Saturate  period=k.Ts  sg_ssr=7*2  UseAsADC=off  ADCChannel='1'  interface=None  automatic_assignment=on  address_offset=hex2dec('00')  intf_name=''  intf_description=''  default_value=0  timing_constraint=None  locs_specified=off  LOCs={}  io_standard={}  inherit_from_input=off  hdl_port=on  interface_prev=1  block_type=realgatewayin_ssr  XmcBlockStatus=1  sg_ssr_prev=14  maskContainerNames=group4  block_width_w=590  block_height_w=670  block_width=640  block_height=850
  LQG_led_in : hdlBasic/Gateway In  gui_display_data_type=Fixed-point  arith_type=Unsigned  n_bits=8  bin_pt=0  preci_type=Single  exp_width=8  frac_width=24  rows=1  columns=1  quantization="Round  (unbiased: +/- Inf)"  overflow=Saturate  period=1  UseAsADC=off  ADCChannel='1'  interface=None  automatic_assignment=on  address_offset=hex2dec('00')  intf_name=''  intf_description=''  default_value=0  timing_constraint=None  locs_specified=off  LOCs={}  io_standard={}  inherit_from_input=off  hdl_port=on  XmcBlockStatus=1  maskContainerNames=group4  block_type=gatewayin  block_config=sysgen:gateway_in_config  block_width_w=590  block_height_w=620  block_width=640  block_height=850
  LQG_led_out : hdlBasic/Gateway Out  inherit_from_input=off  hdl_port=on  rows=1  columns=1  UseAsDAC=off  DACChannel='1'  interface=None  automatic_assignment=on  address_offset=hex2dec('00')  intf_name=''  intf_description=''  timing_constraint=None  locs_specified=off  LOCs={}  io_standard={}  XmcBlockStatus=1  maskContainerNames=group4  block_type=gatewayout  block_config=sysgen:gateway_out_config  block_width_w=590  block_height_w=620  block_width=620  block_height=750
  Terminator : Terminator
  WTF_simulink_get_your_types_correct : hdlSSR/Vector Reinterpret  force_arith_type=on  arith_type="Signed  (2's comp)"  force_bin_pt=on  bin_pt=22  sg_ssr=2  block_type=reinterpret_ssr  XmcBlockStatus=1  sg_ssr_prev=2  maskContainerNames=group1
  accumulate_matmuls : Subsystem
  add_yk_offset : hdlSSR/Vector AddSub Fabric  mode=Addition  use_carryin=off  use_carryout=off  en=off  sg_latency=1  sg_ssr=2  precision=User Defined  arith_type="Signed  (2's comp)"  n_bits=14  bin_pt=12  quantization=Truncate  overflow=Wrap  use_behavioral_HDL=on  hw_selection=Fabric  pipelined=off  block_type=addsub_ssr  XmcBlockStatus=1  sg_ssr_prev=2  maskContainerNames=group1
  add_yk_offset1 : hdlSSR/Vector AddSub Fabric  mode=Addition  use_carryin=off  use_carryout=off  en=off  sg_latency=1  sg_ssr=2  precision=User Defined  arith_type="Signed  (2's comp)"  n_bits=14  bin_pt=12  quantization=Truncate  overflow=Wrap  use_behavioral_HDL=on  hw_selection=Fabric  pipelined=off  block_type=addsub_ssr  XmcBlockStatus=1  sg_ssr_prev=2  maskContainerNames=group1
  cast_2Fix25-22 : hdlSSR/Vector Convert  gui_display_data_type=Fixed-point  arith_type=Signed (2's comp)  n_bits=25  bin_pt=22  float_type=Single  exp_bits=8  fraction_bits=24  quantization=Truncate  overflow=Wrap  en=off  sg_latency=0  sg_ssr=2  pipeline=off  block_type=convert_ssr  XmcBlockStatus=1  sg_ssr_prev=2  maskContainerNames=group2
  conv_uk_14_12 : hdlSSR/Vector Convert  gui_display_data_type=Fixed-point  arith_type=Signed (2's comp)  n_bits=14  bin_pt=12  float_type=Single  exp_bits=8  fraction_bits=24  quantization=Truncate  overflow=Wrap  en=off  sg_latency=0  sg_ssr=2  pipeline=off  block_type=convert_ssr  XmcBlockStatus=1  sg_ssr_prev=2  maskContainerNames=group2
  conv_yk_25_22 : hdlSSR/Vector Convert  gui_display_data_type=Fixed-point  arith_type=Signed (2's comp)  n_bits=25  bin_pt=22  float_type=Single  exp_bits=8  fraction_bits=24  quantization=Truncate  overflow=Wrap  en=off  sg_latency=0  sg_ssr=2  pipeline=off  block_type=convert_ssr  XmcBlockStatus=1  sg_ssr_prev=2  maskContainerNames=group2
  led_inverter : hdlBasic/Inverter  en=off  latency=1  XmcBlockStatus=1  maskContainerNames=group2  block_type=inv  block_config=sysgen:Inverter_config
  matmul_2x7_7x1_0 : Subsystem
  matmul_7x2_2x1_0 : Subsystem
  matmul_7x2_2x1_1 : Subsystem
  matmul_7x7_7x1_0 : Subsystem
  mul_yk_factor : hdlSSR/Vector Real Mult  precision=User Defined  arith_type="Signed  (2's comp)"  n_bits=14  bin_pt=12  quantization=Truncate  overflow=Wrap  en=off  sg_latency=3  sg_ssr=2  use_behavioral_HDL=on  opt=Speed  use_embedded=on  optimum_pipeline=off  pipeline=on  use_rpm=on  placement_style=Triangular  block_type=realmult_ssr  XmcBlockStatus=1  sg_ssr_prev=2  maskContainerNames=group1
  mul_yk_factor1 : hdlSSR/Vector Real Mult  precision=User Defined  arith_type="Signed  (2's comp)"  n_bits=14  bin_pt=12  quantization=Truncate  overflow=Wrap  en=off  sg_latency=3  sg_ssr=2  use_behavioral_HDL=on  opt=Speed  use_embedded=on  optimum_pipeline=off  pipeline=on  use_rpm=on  placement_style=Triangular  block_type=realmult_ssr  XmcBlockStatus=1  sg_ssr_prev=2  maskContainerNames=group1
  repr2vec_2Fix43-37_uk : Subsystem
  repr2vec_7Fix25-22_xkhat : Subsystem
  uk_factor_gw : hdlSSR/Vector Real Gateway In  gui_display_data_type=Fixed-point  arith_type=Signed (2's comp)  n_bits=18  bin_pt=14  preci_type=Single  exp_width=8  frac_width=24  quantization="Round  (unbiased: +/- Inf)"  overflow=Saturate  period=k.Ts  sg_ssr=2  UseAsADC=off  ADCChannel='1'  interface=None  automatic_assignment=on  address_offset=hex2dec('00')  intf_name=''  intf_description=''  default_value=0  timing_constraint=None  locs_specified=off  LOCs={}  io_standard={}  inherit_from_input=off  hdl_port=on  interface_prev=1  block_type=realgatewayin_ssr  XmcBlockStatus=1  sg_ssr_prev=2  maskContainerNames=group4  block_width_w=590  block_height_w=670  block_width=640  block_height=850
  uk_gw : hdlSSR/Vector Real Gateway Out  inherit_from_input=off  hdl_port=on  sg_ssr=2  rows=1  columns=1  UseAsDAC=off  DACChannel='1'  interface=None  automatic_assignment=on  address_offset=hex2dec('00')  intf_name=''  intf_description=''  timing_constraint=None  locs_specified=off  LOCs={}  io_standard={}  block_type=realgatewayout_ssr  XmcBlockStatus=1  sg_ssr_prev=2  maskContainerNames=group4  block_width_w=590  block_height_w=620  block_width=620  block_height=750
  uk_offset_gw : hdlSSR/Vector Real Gateway In  gui_display_data_type=Fixed-point  arith_type=Signed (2's comp)  n_bits=14  bin_pt=12  preci_type=Single  exp_width=8  frac_width=24  quantization="Round  (unbiased: +/- Inf)"  overflow=Saturate  period=k.Ts  sg_ssr=2  UseAsADC=off  ADCChannel='1'  interface=None  automatic_assignment=on  address_offset=hex2dec('00')  intf_name=''  intf_description=''  default_value=0  timing_constraint=None  locs_specified=off  LOCs={}  io_standard={}  inherit_from_input=off  hdl_port=on  interface_prev=1  block_type=realgatewayin_ssr  XmcBlockStatus=1  sg_ssr_prev=2  maskContainerNames=group4  block_width_w=590  block_height_w=670  block_width=640  block_height=850
  vec2repr_14_Gamma_res : Subsystem
  vec2repr_14_Gamma_shift : Subsystem
  vec2repr_14_K_res : Subsystem
  vec2repr_14_K_shift : Subsystem
  vec2repr_14_L_res : Subsystem
  vec2repr_14_L_shift : Subsystem
  vec2repr_2 : Subsystem
  vec2repr_2_uk : Subsystem
  vec2repr_49_F_res : Subsystem
  vec2repr_49_F_shift : Subsystem
  xkhat_gw : hdlSSR/Vector Real Gateway Out  inherit_from_input=off  hdl_port=on  sg_ssr=7  rows=1  columns=1  UseAsDAC=off  DACChannel='1'  interface=None  automatic_assignment=on  address_offset=hex2dec('00')  intf_name=''  intf_description=''  timing_constraint=None  locs_specified=off  LOCs={}  io_standard={}  block_type=realgatewayout_ssr  XmcBlockStatus=1  sg_ssr_prev=7  maskContainerNames=group4  block_width_w=590  block_height_w=620  block_width=620  block_height=750
  yk_factor_gw : hdlSSR/Vector Real Gateway In  gui_display_data_type=Fixed-point  arith_type=Signed (2's comp)  n_bits=18  bin_pt=14  preci_type=Single  exp_width=8  frac_width=24  quantization="Round  (unbiased: +/- Inf)"  overflow=Saturate  period=k.Ts  sg_ssr=2  UseAsADC=off  ADCChannel='1'  interface=None  automatic_assignment=on  address_offset=hex2dec('00')  intf_name=''  intf_description=''  default_value=0  timing_constraint=None  locs_specified=off  LOCs={}  io_standard={}  inherit_from_input=off  hdl_port=on  interface_prev=1  block_type=realgatewayin_ssr  XmcBlockStatus=1  sg_ssr_prev=2  maskContainerNames=group4  block_width_w=590  block_height_w=670  block_width=640  block_height=850
  yk_gw : hdlSSR/Vector Real Gateway In  gui_display_data_type=Fixed-point  arith_type=Signed (2's comp)  n_bits=14  bin_pt=12  preci_type=Single  exp_width=8  frac_width=24  quantization="Round  (unbiased: +/- Inf)"  overflow=Saturate  period=k.Ts  sg_ssr=2  UseAsADC=off  ADCChannel='1'  interface=None  automatic_assignment=on  address_offset=hex2dec('00')  intf_name=''  intf_description=''  default_value=0  timing_constraint=None  locs_specified=off  LOCs={}  io_standard={}  inherit_from_input=off  hdl_port=on  interface_prev=1  block_type=realgatewayin_ssr  XmcBlockStatus=1  sg_ssr_prev=2  maskContainerNames=group4  block_width_w=590  block_height_w=670  block_width=640  block_height=850
  yk_offset_gw : hdlSSR/Vector Real Gateway In  gui_display_data_type=Fixed-point  arith_type=Signed (2's comp)  n_bits=14  bin_pt=12  preci_type=Single  exp_width=8  frac_width=24  quantization="Round  (unbiased: +/- Inf)"  overflow=Saturate  period=k.Ts  sg_ssr=2  UseAsADC=off  ADCChannel='1'  interface=None  automatic_assignment=on  address_offset=hex2dec('00')  intf_name=''  intf_description=''  default_value=0  timing_constraint=None  locs_specified=off  LOCs={}  io_standard={}  inherit_from_input=off  hdl_port=on  interface_prev=1  block_type=realgatewayin_ssr  XmcBlockStatus=1  sg_ssr_prev=2  maskContainerNames=group4  block_width_w=590  block_height_w=670  block_width=640  block_height=850
  Out1 : Outport
  Out2 : Outport  Port=2
  wires:
  vec2repr_2_uk/1(rowmaj_out) -> [u_k]
  matmul_2x7_7x1_0/1(omat) -> repr2vec_2Fix43-37_uk/1(rowmaj_in)
  [xhat_k] -> repr2vec_7Fix25-22_xkhat/1(rowmaj_in)
  LQG_F_shift_gw/1 -> vec2repr_49_F_shift/1(vec_in)
  matmul_7x2_2x1_0/1(omat) -> accumulate_matmuls/2(Gamma*uk)
  accumulate_matmuls/1(Out1) -> Delay/1  "xhat_k1"
  matmul_7x2_2x1_1/1(omat) -> accumulate_matmuls/3(L*yk)
  Delay/1 -> [xhat_k]
  [u_k] -> matmul_7x2_2x1_0/3(rmat)
  cast_2Fix25-22/1 -> WTF_simulink_get_your_types_correct/1
  vec2repr_2/1(rowmaj_out) -> [y_k]
  LQG_K_shift_gw/1 -> vec2repr_14_K_shift/1(vec_in)
  LQG_K_res_gw/1 -> vec2repr_14_K_res/1(vec_in)
  vec2repr_14_Gamma_res/1(rowmaj_out) -> matmul_7x2_2x1_0/1(lmat_residue)
  vec2repr_49_F_res/1(rowmaj_out) -> matmul_7x7_7x1_0/1(lmat_residue)
  WTF_simulink_get_your_types_correct/1 -> conv_uk_14_12/1, vec2repr_2_uk/1(vec_in)
  uk_gw/1 -> Out1/1
  I5/1 -> LQG_Gamma_res_gw/1
  conv_yk_25_22/1 -> vec2repr_2/1(vec_in)
  I6/1 -> LQG_Gamma_shift_gw/1
  I8/1 -> LQG_L_shift_gw/1
  I7/1 -> LQG_L_res_gw/1
  LQG_Gamma_shift_gw/1 -> vec2repr_14_Gamma_shift/1(vec_in)
  I1/1 -> LQG_K_res_gw/1
  vec2repr_49_F_shift/1(rowmaj_out) -> matmul_7x7_7x1_0/2(lmat_shift)
  I3/1 -> LQG_F_res_gw/1
  LQG_Gamma_res_gw/1 -> vec2repr_14_Gamma_res/1(vec_in)
  I4/1 -> LQG_F_shift_gw/1
  I2/1 -> LQG_K_shift_gw/1
  [xhat_k] -> matmul_7x7_7x1_0/3(rmat)
  xkhat_gw/1 -> Out2/1
  [xhat_k] -> matmul_2x7_7x1_0/3(rmat)
  vec2repr_14_L_shift/1(rowmaj_out) -> matmul_7x2_2x1_1/2(lmat_shift)
  repr2vec_2Fix43-37_uk/1(vec_out) -> cast_2Fix25-22/1
  I/1 -> yk_gw/1
  matmul_7x7_7x1_0/1(omat) -> accumulate_matmuls/1(F*xk)
  LQG_F_res_gw/1 -> vec2repr_49_F_res/1(vec_in)
  vec2repr_14_Gamma_shift/1(rowmaj_out) -> matmul_7x2_2x1_0/2(lmat_shift)
  LQG_L_shift_gw/1 -> vec2repr_14_L_shift/1(vec_in)
  vec2repr_14_K_res/1(rowmaj_out) -> matmul_2x7_7x1_0/1(lmat_residue)
  vec2repr_14_L_res/1(rowmaj_out) -> matmul_7x2_2x1_1/1(lmat_residue)
  LQG_L_res_gw/1 -> vec2repr_14_L_res/1(vec_in)
  vec2repr_14_K_shift/1(rowmaj_out) -> matmul_2x7_7x1_0/2(lmat_shift)
  [y_k] -> matmul_7x2_2x1_1/3(rmat)
  yk_gw/1 -> add_yk_offset/1
  add_yk_offset/1 -> mul_yk_factor/1
  mul_yk_factor/1 -> conv_yk_25_22/1
  yk_offset/1 -> yk_offset_gw/1
  yk_factor/1 -> yk_factor_gw/1
  mul_yk_factor1/1 -> add_yk_offset1/1
  conv_uk_14_12/1 -> mul_yk_factor1/1
  add_yk_offset1/1 -> uk_gw/1
  uk_factor/1 -> uk_factor_gw/1
  uk_offset/1 -> uk_offset_gw/1
  repr2vec_7Fix25-22_xkhat/1(vec_out) -> xkhat_gw/1
  yk_offset_gw/1 -> add_yk_offset/2
  yk_factor_gw/1 -> mul_yk_factor/2
  uk_offset_gw/1 -> add_yk_offset1/2
  uk_factor_gw/1 -> mul_yk_factor1/2
  LQG_led_in/1 -> led_inverter/1
  led_inverter/1 -> LQG_led_out/1
  LQG_led_out/1 -> Terminator/1
  Constant/1 -> LQG_led_in/1

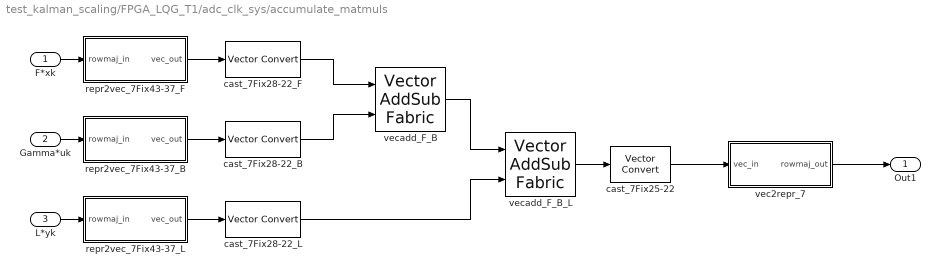
== system test_kalman_scaling/FPGA_LQG_T1/adc_clk_sys/accumulate_matmuls ==
  F*xk : Inport
  Gamma*uk : Inport  Port=2
  L*yk : Inport  Port=3
  cast_7Fix25-22 : hdlSSR/Vector Convert  gui_display_data_type=Fixed-point  arith_type=Signed (2's comp)  n_bits=25  bin_pt=22  float_type=Single  exp_bits=8  fraction_bits=24  quantization=Truncate  overflow=Wrap  en=off  sg_latency=0  sg_ssr=7  pipeline=off  block_type=convert_ssr  XmcBlockStatus=1  sg_ssr_prev=7  maskContainerNames=group2
  cast_7Fix28-22_B : hdlSSR/Vector Convert  gui_display_data_type=Fixed-point  arith_type=Signed (2's comp)  n_bits=28  bin_pt=22  float_type=Single  exp_bits=8  fraction_bits=24  quantization=Truncate  overflow=Wrap  en=off  sg_latency=0  sg_ssr=7  pipeline=off  block_type=convert_ssr  XmcBlockStatus=1  sg_ssr_prev=7  maskContainerNames=group2
  cast_7Fix28-22_F : hdlSSR/Vector Convert  gui_display_data_type=Fixed-point  arith_type=Signed (2's comp)  n_bits=28  bin_pt=22  float_type=Single  exp_bits=8  fraction_bits=24  quantization=Truncate  overflow=Wrap  en=off  sg_latency=0  sg_ssr=7  pipeline=off  block_type=convert_ssr  XmcBlockStatus=1  sg_ssr_prev=7  maskContainerNames=group2
  cast_7Fix28-22_L : hdlSSR/Vector Convert  gui_display_data_type=Fixed-point  arith_type=Signed (2's comp)  n_bits=28  bin_pt=22  float_type=Single  exp_bits=8  fraction_bits=24  quantization=Truncate  overflow=Wrap  en=off  sg_latency=0  sg_ssr=7  pipeline=off  block_type=convert_ssr  XmcBlockStatus=1  sg_ssr_prev=7  maskContainerNames=group2
  repr2vec_7Fix43-37_B : Subsystem
  repr2vec_7Fix43-37_F : Subsystem
  repr2vec_7Fix43-37_L : Subsystem
  vec2repr_7 : Subsystem
  vecadd_F_B : hdlSSR/Vector AddSub Fabric  mode=Addition  use_carryin=off  use_carryout=off  en=off  sg_latency=0  sg_ssr=7  precision=User Defined  arith_type=Unsigned  n_bits=28  bin_pt=22  quantization=Truncate  overflow=Wrap  use_behavioral_HDL=on  hw_selection=Fabric  pipelined=off  block_type=addsub_ssr  XmcBlockStatus=1  sg_ssr_prev=7  maskContainerNames=group1
  vecadd_F_B_L : hdlSSR/Vector AddSub Fabric  mode=Addition  use_carryin=off  use_carryout=off  en=off  sg_latency=0  sg_ssr=7  precision=User Defined  arith_type=Unsigned  n_bits=28  bin_pt=22  quantization=Truncate  overflow=Wrap  use_behavioral_HDL=on  hw_selection=Fabric  pipelined=off  block_type=addsub_ssr  XmcBlockStatus=1  sg_ssr_prev=7  maskContainerNames=group1
  Out1 : Outport
  wires:
  F*xk/1 -> repr2vec_7Fix43-37_F/1(rowmaj_in)
  Gamma*uk/1 -> repr2vec_7Fix43-37_B/1(rowmaj_in)
  L*yk/1 -> repr2vec_7Fix43-37_L/1(rowmaj_in)
  repr2vec_7Fix43-37_F/1(vec_out) -> cast_7Fix28-22_F/1
  repr2vec_7Fix43-37_B/1(vec_out) -> cast_7Fix28-22_B/1
  cast_7Fix28-22_F/1 -> vecadd_F_B/1
  cast_7Fix28-22_B/1 -> vecadd_F_B/2
  repr2vec_7Fix43-37_L/1(vec_out) -> cast_7Fix28-22_L/1
  vecadd_F_B/1 -> vecadd_F_B_L/1
  cast_7Fix28-22_L/1 -> vecadd_F_B_L/2
  vecadd_F_B_L/1 -> cast_7Fix25-22/1
  cast_7Fix25-22/1 -> vec2repr_7/1(vec_in)
  vec2repr_7/1(rowmaj_out) -> Out1/1

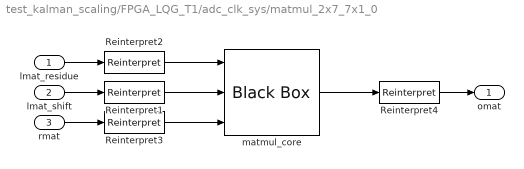
== system test_kalman_scaling/FPGA_LQG_T1/adc_clk_sys/matmul_2x7_7x1_0 ==
  lmat_residue : Inport
  lmat_shift : Inport  Port=2
  rmat : Inport  Port=3
  Reinterpret{1..4} (4 alike) : hdlBasic/Reinterpret  force_arith_type=on  arith_type=Unsigned  force_bin_pt=on  bin_pt=0  XmcBlockStatus=1  maskContainerNames=group1  block_type=reinterpret  block_config=sysgen:Reinterpret_config
  matmul_core : hdlBasic/Black Box  init_code=matmul_shiftfix_2x7_7x1  sim_method=Vivado Simulator  verbose=off  XmcBlockStatus=1  maskContainerNames=group1  block_type=blackbox2  block_config=sysgen:black_box_config
  omat : Outport
  wires:
  rmat/1 -> Reinterpret3/1
  lmat_shift/1 -> Reinterpret1/1
  lmat_residue/1 -> Reinterpret2/1
  matmul_core/1 -> Reinterpret4/1
  Reinterpret2/1 -> matmul_core/1
  Reinterpret1/1 -> matmul_core/2
  Reinterpret3/1 -> matmul_core/3
  Reinterpret4/1 -> omat/1

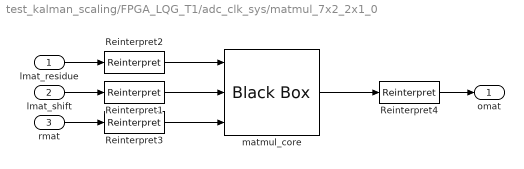
== system test_kalman_scaling/FPGA_LQG_T1/adc_clk_sys/matmul_7x2_2x1_0 ==
  lmat_residue : Inport
  lmat_shift : Inport  Port=2
  rmat : Inport  Port=3
  Reinterpret{1..4} (4 alike) : hdlBasic/Reinterpret  force_arith_type=on  arith_type=Unsigned  force_bin_pt=on  bin_pt=0  XmcBlockStatus=1  maskContainerNames=group1  block_type=reinterpret  block_config=sysgen:Reinterpret_config
  matmul_core : hdlBasic/Black Box  init_code=matmul_shiftfix_7x2_2x1  sim_method=Vivado Simulator  verbose=off  XmcBlockStatus=1  maskContainerNames=group1  block_type=blackbox2  block_config=sysgen:black_box_config
  omat : Outport
  wires:
  rmat/1 -> Reinterpret3/1
  lmat_shift/1 -> Reinterpret1/1
  lmat_residue/1 -> Reinterpret2/1
  matmul_core/1 -> Reinterpret4/1
  Reinterpret2/1 -> matmul_core/1
  Reinterpret1/1 -> matmul_core/2
  Reinterpret3/1 -> matmul_core/3
  Reinterpret4/1 -> omat/1

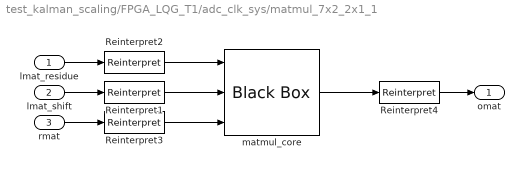
== system test_kalman_scaling/FPGA_LQG_T1/adc_clk_sys/matmul_7x2_2x1_1 ==
  lmat_residue : Inport
  lmat_shift : Inport  Port=2
  rmat : Inport  Port=3
  Reinterpret{1..4} (4 alike) : hdlBasic/Reinterpret  force_arith_type=on  arith_type=Unsigned  force_bin_pt=on  bin_pt=0  XmcBlockStatus=1  maskContainerNames=group1  block_type=reinterpret  block_config=sysgen:Reinterpret_config
  matmul_core : hdlBasic/Black Box  init_code=matmul_shiftfix_7x2_2x1  sim_method=Vivado Simulator  verbose=off  XmcBlockStatus=1  maskContainerNames=group1  block_type=blackbox2  block_config=sysgen:black_box_config
  omat : Outport
  wires:
  rmat/1 -> Reinterpret3/1
  lmat_shift/1 -> Reinterpret1/1
  lmat_residue/1 -> Reinterpret2/1
  matmul_core/1 -> Reinterpret4/1
  Reinterpret2/1 -> matmul_core/1
  Reinterpret1/1 -> matmul_core/2
  Reinterpret3/1 -> matmul_core/3
  Reinterpret4/1 -> omat/1

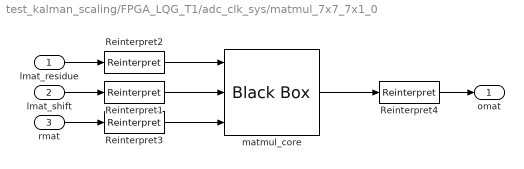
== system test_kalman_scaling/FPGA_LQG_T1/adc_clk_sys/matmul_7x7_7x1_0 ==
  lmat_residue : Inport
  lmat_shift : Inport  Port=2
  rmat : Inport  Port=3
  Reinterpret{1..4} (4 alike) : hdlBasic/Reinterpret  force_arith_type=on  arith_type=Unsigned  force_bin_pt=on  bin_pt=0  XmcBlockStatus=1  maskContainerNames=group1  block_type=reinterpret  block_config=sysgen:Reinterpret_config
  matmul_core : hdlBasic/Black Box  init_code=matmul_shiftfix_7x7_7x1  sim_method=Vivado Simulator  verbose=off  XmcBlockStatus=1  maskContainerNames=group1  block_type=blackbox2  block_config=sysgen:black_box_config
  omat : Outport
  wires:
  rmat/1 -> Reinterpret3/1
  lmat_shift/1 -> Reinterpret1/1
  lmat_residue/1 -> Reinterpret2/1
  matmul_core/1 -> Reinterpret4/1
  Reinterpret2/1 -> matmul_core/1
  Reinterpret1/1 -> matmul_core/2
  Reinterpret3/1 -> matmul_core/3
  Reinterpret4/1 -> omat/1
